simulink model "Q_2_1_2_2_SSC_Robust_Tracking_DISCRETE"  (R2024b)
settings: Solver=VariableStepAuto  StartTime=0.0  StopTime=10  FixedStep=0.001  RelTol=1e-3
values from neighbouring files (symbols this model uses):
  delta_c = 1 / sqrt(2)    [SS_Calculations.m]    (also in plant_calculations.m)
  Gamma_o = [Gamma2 - L*Gamma1, (Phi22 - L*Phi12)*L + Phi21 - L*Phi11]    [Q1_2_2_2_Direct_digital_design.m]
  H_o = [0 1]    [Q1_2_2_2_Direct_digital_design.m]
  J_o = [0 1; 0 L]    [Q1_2_2_2_Direct_digital_design.m]
  K_W = 1 / T_W    (= 71.4285714286)    [plant_calculations.m]
  Nr = Nu + K*Nx    [Q1_2.2.2(part2)_Direct_digital_design.m]    (also in SS_nominal_tracking.m = Nu + K * Nx)
  Nu = sol(3)    [Q1_2.2.2(part2)_Direct_digital_design.m]    (also in SS_nominal_tracking.m)
  Nx = sol(1:2)    [Q1_2.2.2(part2)_Direct_digital_design.m]    (also in SS_nominal_tracking.m)
  Phi_o = Phi22 - L * Phi12    [Q1_2_2_2_Direct_digital_design.m]
  T_sample = 1e-3    (= 0.001)    [discrete_time_basics.m]
  w_c = 2 * pi * 50    (= 314.159265359)    [SS_Calculations.m]    (also in plant_calculations.m = 125.663706144)
undefined symbols (not defined in the file or in its folder): DiscIntNeverNeededParam, gbox, K_e, KI_e, rads2rpm, sens
libraries: simulink x2
settings Model: Creator=JS  LastModifiedBy=JS

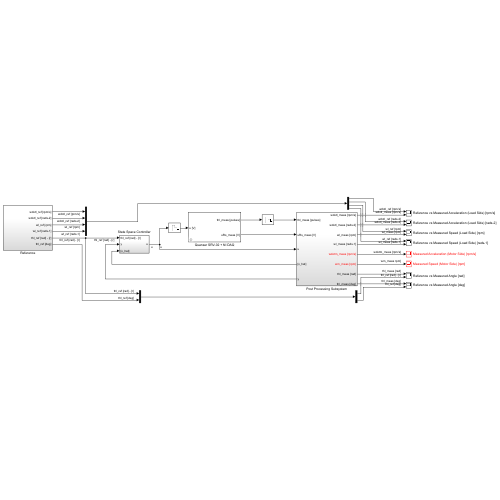
[thumbnail: Simulink's stored preview of the top-level diagram]
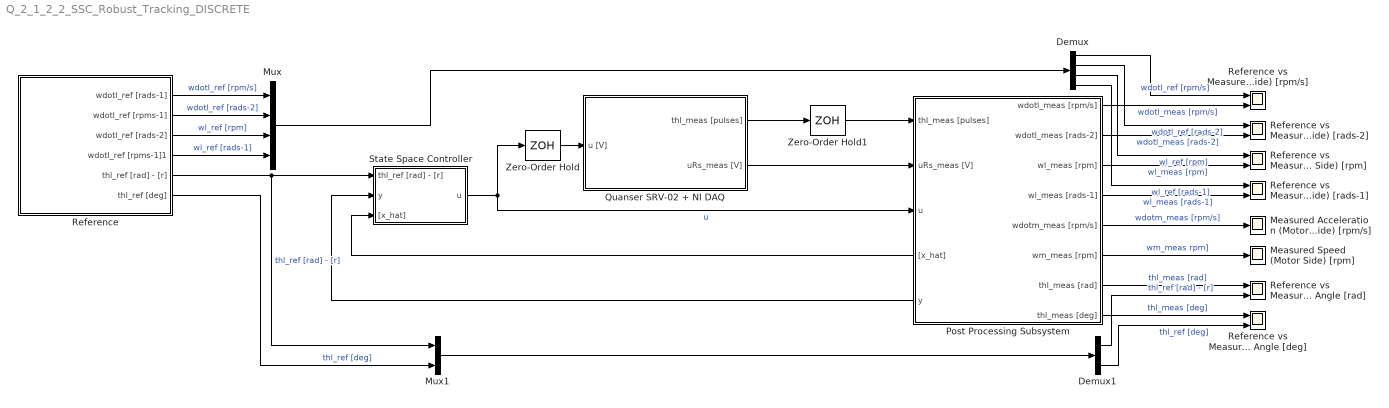
== system Q_2_1_2_2_SSC_Robust_Tracking_DISCRETE ==
  Demux : Demux
  Demux1 : Demux  Outputs=2
  Measured Acceleration (Motor Side) [rpm/s] : Scope
  Measured Speed (Motor Side) [rpm] : Scope
  Mux : Mux
  Mux1 : Mux  Inputs=2
  Post Processing Subsystem : Subsystem
      settings: PortSchema="{\"entries\":[{\"content\":{\"sides\":[{\"content\":{\"connectorIds\":[\"In1\",\"In2\",\"In3\",\"Out9\",\"Out10\"]},\"type\":\"ConnectorPlacement.EquallySpacedRectSide\",\"uuid\":\"6767711d-56d4-4572-b74d-4fb019252509\"},{\"content\":{\"connectorIds\":[\"Out1\",\"Out2\",\"Out3\",\"Out4\",\"Out5\",\"Out6\",\"Out7\",\"Out8\"],\"side\":\"RIGHT\"},\"type\":\"ConnectorPlacement.EquallySpacedRectSide\",\"uuid\":\"a9f5ae09-2012-4431-ba40-a840a86176f2\"},{\"content\":{\"side\":\"TOP\"},\"type\":\"ConnectorPlacement.EquallySpacedRectSide\",\"uuid\":\"770e752c-ca34-4fe9-9680-0253f89658d7\"}]},\"type\":\"ConnectorPlacement.EquallySpacedConnector\",\"uuid\":\"ae0efa9d-d1b9-4714-bd70-449b4c0cafd2\"}],\"packageUris\":[\"http://schema.mathworks.com/mf0/Connector/R2020b\"],\"version\":\"1.0\"}"
  Quanser SRV-02 + NI DAQ : Subsystem  mask(Quanser SRV-02 (with inertial load) + NI DAQ){Ts=0.001, fricType=Coulomb + viscous}
      mask prompts: Ts "NI DAQ Sample Time:"; fricType "Friction model"
      mask help: Quanser SRV-02 (with inertial load) + NI DAQ model.
      mask init:
      | %%  Sensors data
      | 
      | %   shunt resistor
      | sens.curr.Rs = 0.5;                         %   resistance [Ohm]   
      | sens.curr.uRs_std = 0.01;                   %   voltage noise standard dev [V]                           
      | sens.curr.uRs_var = sens.curr.uRs_std^2;	%   voltage noise variance [V^2]
      | 
      | %   Hewlett-Packard HEDS-5540#A06 optical encoder
      | sens.enc.ppr = 500*4;                       %   pulses per rotation
      | sens.enc.pulse2deg = 360/sens.enc.ppr;      %   [pulses] -> [deg]
      | sens.enc.pulse2rad = 2*pi/sens.enc.ppr;     %   [pulses] -> [rad]
      | sens.enc.deg2pulse = sens.enc.ppr/360;      %   [deg] -> [pulses]
      | sens.enc.rad2pulse = sens.enc.ppr/2/pi;     %   [rad] -> [pulses]
      | 
      | 
      | %%  Data acquisition board (daq) data
      | 
      | %   NI PCI-6221 DAC data
      | daq.dac.bits = 16;                                  %   resolution (bits)
      | daq.dac.fs   = 10;                                  %   full scale 
      | daq.dac.q    = 2*daq.dac.fs/(2^daq.dac.bits-1);     %	quantization
      | 
      | %   NI PCI-6221 ADC data
      | daq.adc.bits = 16;                                  %   resolution (bits)
      | daq.adc.fs   = 10;                                  %   full scale (as set in SLDRT Analog Input block)
      | daq.adc.q    = 2*daq.adc.fs/(2^daq.adc.bits-1);     %   quantization
      mask Help:
      | Riccardo Antonello (antonello@dei.unipd.it)
      | 
      | April 24, 2020
      | 
      | Dept. of Information Engineering, University of Padova
      mask TypeOptions fricType: Coulomb + viscous | Karnopp
  Reference : Subsystem
  Reference vs Measured Acceleration (Load Side) [rads-2] : Scope  NumInputPorts=2
  Reference vs Measured Acceleration (Load Side) [rpm/s] : Scope  NumInputPorts=2
  "Reference vs Measured Angle [deg] " : Scope  NumInputPorts=2
  "Reference vs Measured Angle [rad] " : Scope  NumInputPorts=2
  Reference vs Measured Speed (Load Side) [rads-1] : Scope  NumInputPorts=2
  Reference vs Measured Speed (Load Side) [rpm] : Scope  NumInputPorts=2
  State Space Controller : Subsystem
  Zero-Order Hold : ZeroOrderHold  SampleTime=T_sample
  Zero-Order Hold1 : ZeroOrderHold  SampleTime=T_sample
  wires:
  Reference/5(thl_ref [rad] - [r]) -> Mux1/1, State Space Controller/1(thl_ref [rad] - [r])  "thl_ref [rad] - [r]"
  Reference/2(wdotl_ref [rpms-1]) -> Mux/2  "wdotl_ref [rads-2]"
  Reference/1(wdotl_ref [rads-1]) -> Mux/1  "wdotl_ref [rpm/s]"
  Reference/6(thl_ref [deg]) -> Mux1/2  "thl_ref [deg]"
  State Space Controller/1(u) -> Zero-Order Hold/1, Post Processing Subsystem/3(u)  "u"
  Quanser SRV-02 + NI DAQ/2(uRs_meas [V]) -> Post Processing Subsystem/2(uRs_meas [V])
  Post Processing Subsystem/1(wdotl_meas [rpm/s]) -> Reference vs Measured Acceleration (Load Side) [rpm/s]/2  "wdotl_meas [rpm/s]"
  Post Processing Subsystem/8(thl_meas [deg]) -> "Reference vs Measured Angle [deg] "/1  "thl_meas [deg]"
  Post Processing Subsystem/7(thl_meas [rad]) -> "Reference vs Measured Angle [rad] "/1  "thl_meas [rad]"
  Post Processing Subsystem/2(wdotl_meas [rads-2]) -> Reference vs Measured Acceleration (Load Side) [rads-2]/2  "wdotl_meas [rads-2]"
  Post Processing Subsystem/9("[x_hat]") -> State Space Controller/3("[x_hat]")
  Post Processing Subsystem/5(wdotm_meas [rpm/s]) -> Measured Acceleration (Motor Side) [rpm/s]/1  "wdotm_meas [rpm/s]"
  Post Processing Subsystem/6(wm_meas [rpm]) -> Measured Speed (Motor Side) [rpm]/1  "wm_meas rpm]"
  Post Processing Subsystem/4(wl_meas [rads-1]) -> Reference vs Measured Speed (Load Side) [rads-1]/2  "wl_meas [rads-1]"
  Post Processing Subsystem/3(wl_meas [rpm]) -> Reference vs Measured Speed (Load Side) [rpm]/2  "wl_meas [rpm]"
  Reference/3(wdotl_ref [rads-2]) -> Mux/3  "wl_ref [rpm]"
  Reference/4(wdotl_ref [rpms-1]1) -> Mux/4  "wl_ref [rads-1]"
  Demux/1 -> Reference vs Measured Acceleration (Load Side) [rpm/s]/1  "wdotl_ref [rpm/s]"
  Demux/2 -> Reference vs Measured Acceleration (Load Side) [rads-2]/1  "wdotl_ref [rads-2]"
  Demux/3 -> Reference vs Measured Speed (Load Side) [rpm]/1  "wl_ref [rpm]"
  Demux/4 -> Reference vs Measured Speed (Load Side) [rads-1]/1  "wl_ref [rads-1]"
  Mux/1 -> Demux/1
  Mux1/1 -> Demux1/1
  Demux1/1 -> "Reference vs Measured Angle [rad] "/2  "thl_ref [rad] - [r]"
  Demux1/2 -> "Reference vs Measured Angle [deg] "/2  "thl_ref [deg]"
  Quanser SRV-02 + NI DAQ/1(thl_meas [pulses]) -> Zero-Order Hold1/1
  Zero-Order Hold/1 -> Quanser SRV-02 + NI DAQ/1(u [V])
  Zero-Order Hold1/1 -> Post Processing Subsystem/1(thl_meas [pulses])
  Post Processing Subsystem/10(y) -> State Space Controller/2(y)

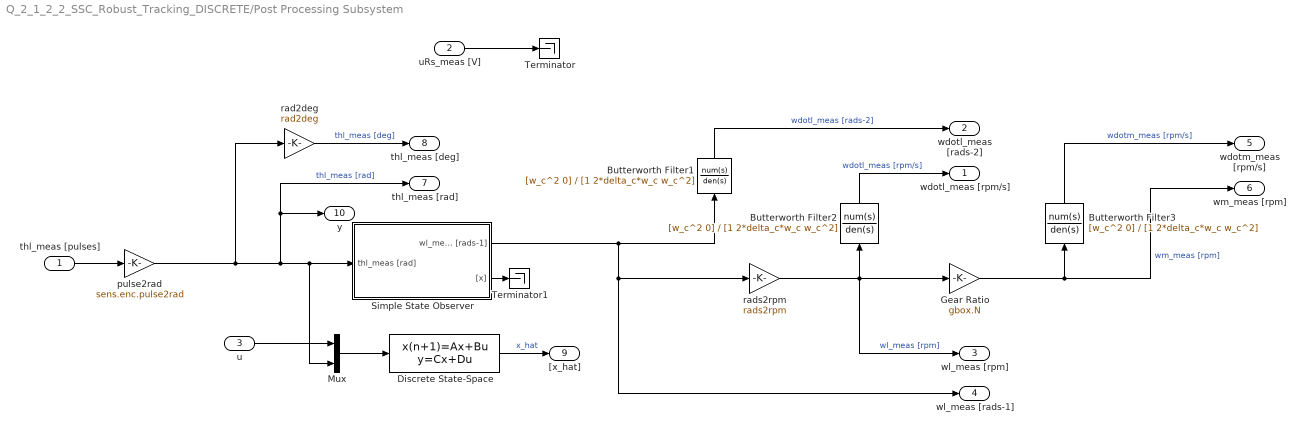
== system Q_2_1_2_2_SSC_Robust_Tracking_DISCRETE/Post Processing Subsystem ==
  thl_meas [pulses] : Inport
  uRs_meas [V] : Inport  Port=2
  u : Inport  Port=3
  Butterworth Filter1 : TransferFcn  Numerator=[w_c^2 0]  Denominator=[1 2*delta_c*w_c w_c^2]
  Butterworth Filter2 : TransferFcn  Numerator=[w_c^2 0]  Denominator=[1 2*delta_c*w_c w_c^2]
  Butterworth Filter3 : TransferFcn  Numerator=[w_c^2 0]  Denominator=[1 2*delta_c*w_c w_c^2]
  Discrete State-Space : DiscreteStateSpace  A=Phi_o  B=Gamma_o  C=H_o  D=J_o  SampleTime=T_sample
  Gear Ratio : Gain  Gain=gbox.N
  Mux : Mux  Inputs=2
  Simple State Observer : Subsystem
  Terminator : Terminator
  Terminator1 : Terminator
  pulse2rad : Gain  Gain=sens.enc.pulse2rad
  rad2deg : Gain  Gain=rad2deg
  rads2rpm : Gain  Gain=rads2rpm
  wdotl_meas [rpm/s] : Outport
  wdotl_meas [rads-2] : Outport  Port=2
  wl_meas [rpm] : Outport  Port=3
  wl_meas [rads-1] : Outport  Port=4
  wdotm_meas [rpm/s] : Outport  Port=5
  wm_meas [rpm] : Outport  Port=6
  thl_meas [rad] : Outport  Port=7
  thl_meas [deg] : Outport  Port=8
  "[x_hat]" : Outport  Port=9
  y : Outport  Port=10
  wires:
  pulse2rad/1 -> Mux/2, Simple State Observer/1(thl_meas [rad]), y/1, thl_meas [rad]/1, rad2deg/1  "thl_meas [rad]"
  rad2deg/1 -> thl_meas [deg]/1  "thl_meas [deg]"
  uRs_meas [V]/1 -> Terminator/1
  thl_meas [pulses]/1 -> pulse2rad/1
  Butterworth Filter3/1 -> wdotm_meas [rpm/s]/1  "wdotm_meas [rpm/s]"
  Butterworth Filter2/1 -> wdotl_meas [rpm/s]/1  "wdotl_meas [rpm/s]"
  rads2rpm/1 -> Gear Ratio/1, wl_meas [rpm]/1, Butterworth Filter2/1  "wl_meas [rpm]"
  Butterworth Filter1/1 -> wdotl_meas [rads-2]/1  "wdotl_meas [rads-2]"
  Gear Ratio/1 -> wm_meas [rpm]/1, Butterworth Filter3/1  "wm_meas [rpm]"
  Simple State Observer/1(wl_meas [rads-1]) -> Butterworth Filter1/1, rads2rpm/1, wl_meas [rads-1]/1
  Simple State Observer/2("[x]") -> Terminator1/1
  Mux/1 -> Discrete State-Space/1
  u/1 -> Mux/1
  Discrete State-Space/1 -> "[x_hat]"/1  "x_hat"

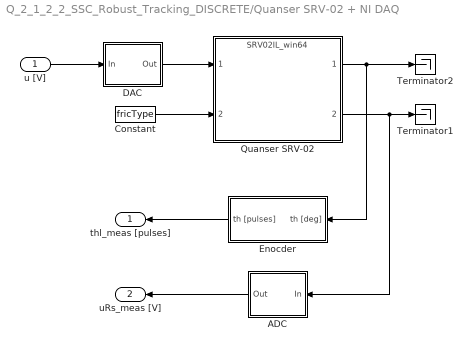
== system Q_2_1_2_2_SSC_Robust_Tracking_DISCRETE/Quanser SRV-02 + NI DAQ ==
  u [V] : Inport
  ADC : Subsystem
  Constant : Constant  Value=fricType
  DAC : Subsystem
  Enocder : Subsystem
  Quanser SRV-02 : ModelReference  ModelNameDialog=SRV02IL_win64.slxp  ModelReferenceVersion=1.44  CopyOfModelProtected=on
  Terminator1 : Terminator
  Terminator2 : Terminator
  thl_meas [pulses] : Outport
  uRs_meas [V] : Outport  Port=2
  wires:
  Enocder/1(th [pulses]) -> thl_meas [pulses]/1
  ADC/1(Out) -> uRs_meas [V]/1
  DAC/1(Out) -> Quanser SRV-02/1
  Quanser SRV-02/2 -> ADC/1(In), Terminator1/1
  u [V]/1 -> DAC/1(In)
  Quanser SRV-02/1 -> Enocder/1(th [deg]), Terminator2/1
  Constant/1 -> Quanser SRV-02/2

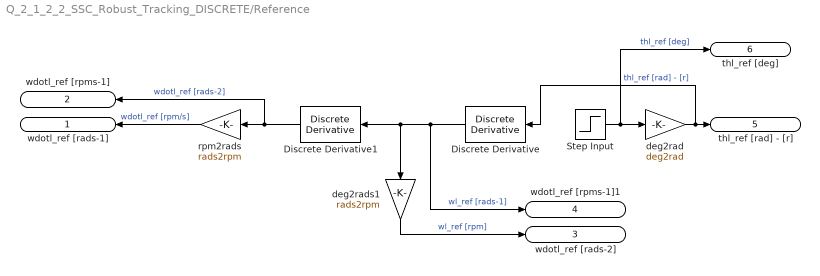
== system Q_2_1_2_2_SSC_Robust_Tracking_DISCRETE/Reference ==
  Discrete Derivative : simulink/Discrete/Discrete Derivative  gainval=1.0  ICPrevScaledInput=0.0  OutMin=[]  OutMax=[]  OutDataType=fixdt(1, 16)  OutScaling=2^-10  DoSatur=off
  Discrete Derivative1 : simulink/Discrete/Discrete Derivative  gainval=1.0  ICPrevScaledInput=0.0  OutMin=[]  OutMax=[]  OutDataType=fixdt(1, 16)  OutScaling=2^-10  DoSatur=off
  Step Input : Step  Time=0  After=70  SampleTime=0
  deg2rad : Gain  Gain=deg2rad
  deg2rads1 : Gain  Gain=rads2rpm
  rpm2rads : Gain  Gain=rads2rpm
  wdotl_ref [rads-1] : Outport
  wdotl_ref [rpms-1] : Outport  Port=2
  wdotl_ref [rads-2] : Outport  Port=3
  wdotl_ref [rpms-1]1 : Outport  Port=4
  thl_ref [rad] - [r] : Outport  Port=5
  thl_ref [deg] : Outport  Port=6
  wires:
  deg2rad/1 -> Discrete Derivative/1, thl_ref [rad] - [r]/1  "thl_ref [rad] - [r]"
  Step Input/1 -> thl_ref [deg]/1, deg2rad/1  "thl_ref [deg]"
  Discrete Derivative1/1 -> rpm2rads/1, wdotl_ref [rpms-1]/1  "wdotl_ref [rads-2]"
  rpm2rads/1 -> wdotl_ref [rads-1]/1  "wdotl_ref [rpm/s]"
  Discrete Derivative/1 -> Discrete Derivative1/1, deg2rads1/1, wdotl_ref [rpms-1]1/1  "wl_ref [rads-1]"
  deg2rads1/1 -> wdotl_ref [rads-2]/1  "wl_ref [rpm]"

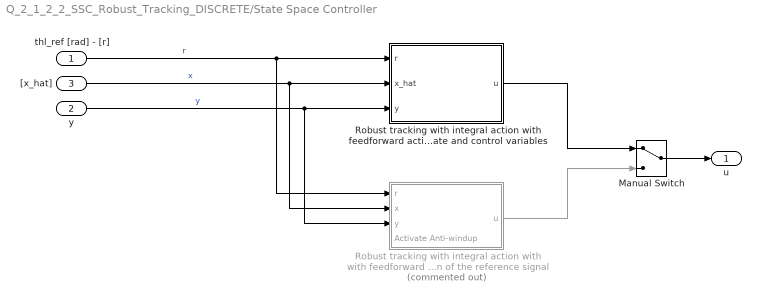
== system Q_2_1_2_2_SSC_Robust_Tracking_DISCRETE/State Space Controller ==
  thl_ref [rad] - [r] : Inport
  y : Inport  Port=2
  "[x_hat]" : Inport  Port=3
  "  Robust tracking with integral action with feedforward action on state and control variables" : Subsystem
  " Robust tracking with integral action with with feedforward compensation of the reference signal" : Subsystem  Commented=on
  Manual Switch : ManualSwitch
  u : Outport
  wires:
  Manual Switch/1 -> u/1
  thl_ref [rad] - [r]/1 -> "  Robust tracking with integral action with feedforward action on state and control variables"/1(r), " Robust tracking with integral action with with feedforward compensation of the reference signal"/1(r)  "r"
  y/1 -> " Robust tracking with integral action with with feedforward compensation of the reference signal"/3(y), "  Robust tracking with integral action with feedforward action on state and control variables"/3(y)  "y"
  "  Robust tracking with integral action with feedforward action on state and control variables"/1(u) -> Manual Switch/1
  "[x_hat]"/1 -> " Robust tracking with integral action with with feedforward compensation of the reference signal"/2(x), "  Robust tracking with integral action with feedforward action on state and control variables"/2(x_hat)  "x"
  " Robust tracking with integral action with with feedforward compensation of the reference signal"/1(u) -> Manual Switch/2

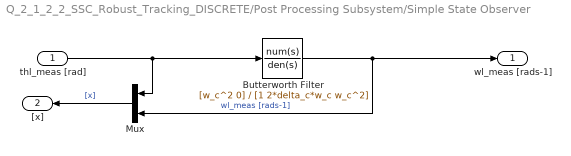
== system Q_2_1_2_2_SSC_Robust_Tracking_DISCRETE/Post Processing Subsystem/Simple State Observer ==
  thl_meas [rad] : Inport
  Butterworth Filter : TransferFcn  Numerator=[w_c^2 0]  Denominator=[1 2*delta_c*w_c w_c^2]
  Mux : Mux  Inputs=2
  wl_meas [rads-1] : Outport
  "[x]" : Outport  Port=2
  wires:
  thl_meas [rad]/1 -> Butterworth Filter/1, Mux/1
  Butterworth Filter/1 -> wl_meas [rads-1]/1, Mux/2  "wl_meas [rads-1]"
  Mux/1 -> "[x]"/1  "[x]"

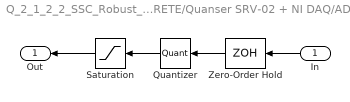
== system Q_2_1_2_2_SSC_Robust_Tracking_DISCRETE/Quanser SRV-02 + NI DAQ/ADC ==
  In : Inport
  Quantizer : Quantizer  QuantizationInterval=daq.adc.q
  Saturation : Saturate  UpperLimit=daq.adc.fs  LowerLimit=-daq.adc.fs
  Zero-Order Hold : ZeroOrderHold  SampleTime=Ts
  Out : Outport
  wires:
  Saturation/1 -> Out/1
  In/1 -> Zero-Order Hold/1
  Quantizer/1 -> Saturation/1
  Zero-Order Hold/1 -> Quantizer/1

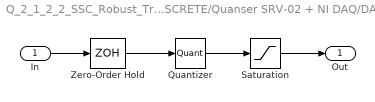
== system Q_2_1_2_2_SSC_Robust_Tracking_DISCRETE/Quanser SRV-02 + NI DAQ/DAC ==
  In : Inport
  Quantizer : Quantizer  QuantizationInterval=daq.dac.q
  Saturation : Saturate  UpperLimit=daq.dac.fs  LowerLimit=-daq.dac.fs
  Zero-Order Hold : ZeroOrderHold  SampleTime=Ts
  Out : Outport
  wires:
  Quantizer/1 -> Saturation/1
  In/1 -> Zero-Order Hold/1
  Zero-Order Hold/1 -> Quantizer/1
  Saturation/1 -> Out/1

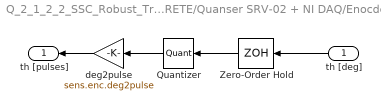
== system Q_2_1_2_2_SSC_Robust_Tracking_DISCRETE/Quanser SRV-02 + NI DAQ/Enocder ==
  th [deg] : Inport
  Quantizer : Quantizer  QuantizationInterval=sens.enc.pulse2deg
  Zero-Order Hold : ZeroOrderHold  SampleTime=Ts
  deg2pulse : Gain  Gain=sens.enc.deg2pulse
  th [pulses] : Outport
  wires:
  Quantizer/1 -> deg2pulse/1
  th [deg]/1 -> Zero-Order Hold/1
  Zero-Order Hold/1 -> Quantizer/1
  deg2pulse/1 -> th [pulses]/1

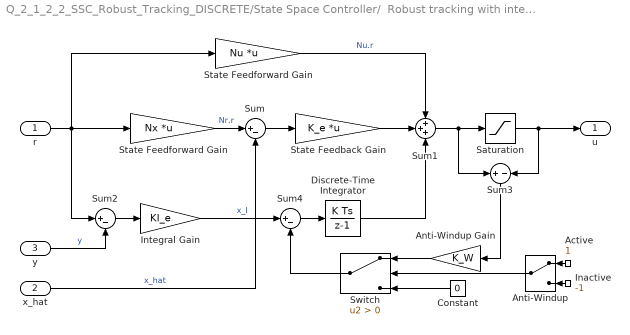
== system Q_2_1_2_2_SSC_Robust_Tracking_DISCRETE/State Space Controller/  Robust tracking with integral action with feedforward action on state and control variables ==
  r : Inport
  x_hat : Inport  Port=2
  y : Inport  Port=3
  Active : Constant
  Anti-Windup : ManualSwitch
  Anti-Windup Gain : Gain  Gain=K_W
  Constant : Constant  Value=0
  Discrete-Time Integrator : DiscreteIntegrator  gainval=K_sample  SampleTime=T_sample  ICPrevOutput=DiscIntNeverNeededParam  ICPrevScaledInput=DiscIntNeverNeededParam
  Inactive : Constant  Value=-1
  Integral Gain : Gain  Gain=KI_e
  Saturation : Saturate  UpperLimit=10  LowerLimit=-10  LinearizeAsGain=off  ZeroCross=off
  State Feedback Gain : Gain  Gain=K_e  Multiplication=Matrix(K*u) (u vector)
  State Feedforward Gain : Gain  Gain=Nx  Multiplication=Matrix(K*u) (u vector)
  "State Feedforward Gain   " : Gain  Gain=Nu  Multiplication=Matrix(K*u) (u vector)
  Sum : Sum  Inputs=|+-
  Sum1 : Sum  Inputs=+++
  Sum2 : Sum  Inputs=|+-
  Sum3 : Sum  Inputs=+|-
  Sum4 : Sum  Inputs=|+-
  Switch : Switch  Criteria=u2 > Threshold  SaturateOnIntegerOverflow=off  InputSameDT=off
  u : Outport
  wires:
  r/1 -> "State Feedforward Gain   "/1, State Feedforward Gain/1, Sum2/1
  State Feedforward Gain/1 -> Sum/1  "Nr.r"
  x_hat/1 -> Sum/2  "x_hat"
  Integral Gain/1 -> Sum4/1  "x_I"
  y/1 -> Sum2/2  "y"
  Sum2/1 -> Integral Gain/1
  Sum1/1 -> Saturation/1, Sum3/1
  Sum3/1 -> Anti-Windup Gain/1
  Anti-Windup/1 -> Switch/2
  Constant/1 -> Switch/3
  Switch/1 -> Sum4/2
  Saturation/1 -> u/1, Sum3/2
  Anti-Windup Gain/1 -> Switch/1
  Sum4/1 -> Discrete-Time Integrator/1
  Inactive/1 -> Anti-Windup/2
  Active/1 -> Anti-Windup/1
  Sum/1 -> State Feedback Gain/1
  Discrete-Time Integrator/1 -> Sum1/3
  State Feedback Gain/1 -> Sum1/2
  "State Feedforward Gain   "/1 -> Sum1/1  "Nu.r"

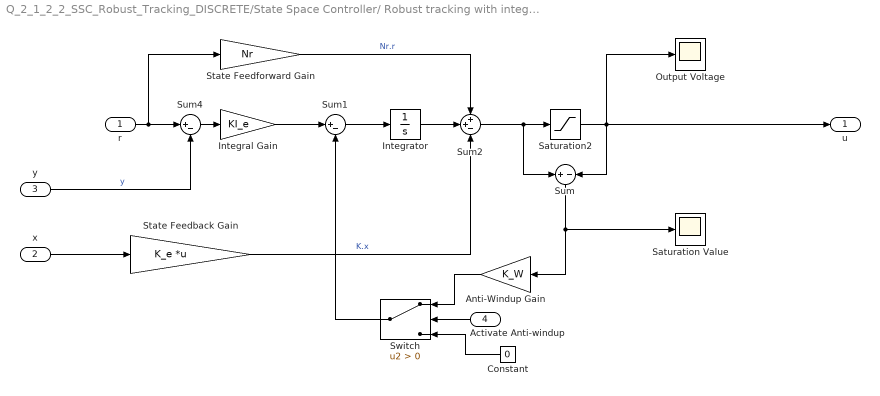
== system Q_2_1_2_2_SSC_Robust_Tracking_DISCRETE/State Space Controller/ Robust tracking with integral action with with feedforward compensation of the reference signal ==
  r : Inport
  x : Inport  Port=2
  y : Inport  Port=3
  Activate Anti-windup : Inport  Port=4
  Anti-Windup Gain : Gain  Gain=K_W
  Constant : Constant  Value=0
  Integral Gain : Gain  Gain=KI_e
  "Integrator " : Integrator
  Output Voltage : Scope
  Saturation Value : Scope
  Saturation2 : Saturate  UpperLimit=10  LowerLimit=-10
  State Feedback Gain : Gain  Gain=K_e  Multiplication=Matrix(K*u) (u vector)
  State Feedforward Gain : Gain  Gain=Nr
  Sum : Sum  Inputs=+|-
  Sum1 : Sum  Inputs=|+-
  Sum2 : Sum  Inputs=++-
  Sum4 : Sum  Inputs=|+-
  Switch : Switch  Criteria=u2 > Threshold  SaturateOnIntegerOverflow=off  InputSameDT=off
  u : Outport
  wires:
  State Feedback Gain/1 -> Sum2/3  "K.x"
  State Feedforward Gain/1 -> Sum2/1  "Nr.r"
  x/1 -> State Feedback Gain/1
  r/1 -> Sum4/1, State Feedforward Gain/1
  Integral Gain/1 -> Sum1/1
  "Integrator "/1 -> Sum2/2
  Sum4/1 -> Integral Gain/1
  y/1 -> Sum4/2  "y"
  Saturation2/1 -> Sum/2, Output Voltage/1, u/1
  Sum2/1 -> Sum/1, Saturation2/1
  Sum/1 -> Anti-Windup Gain/1, Saturation Value/1
  Anti-Windup Gain/1 -> Switch/1
  Constant/1 -> Switch/3
  Activate Anti-windup/1 -> Switch/2
  Switch/1 -> Sum1/2
  Sum1/1 -> "Integrator "/1
